simulink model "Solar_Panel_Tracker"  (R2024a)
settings: Solver=VariableStepAuto  StartTime=0.0  StopTime=10.0  RelTol=1e-3
settings Model: Creator=VICTUS  LastModifiedBy=VICTUS

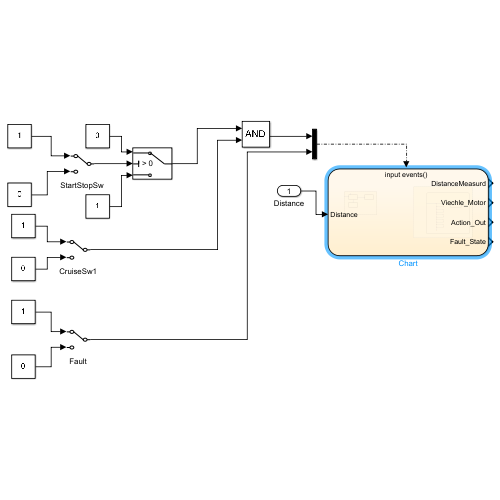
[thumbnail: Simulink's stored preview of the top-level diagram]
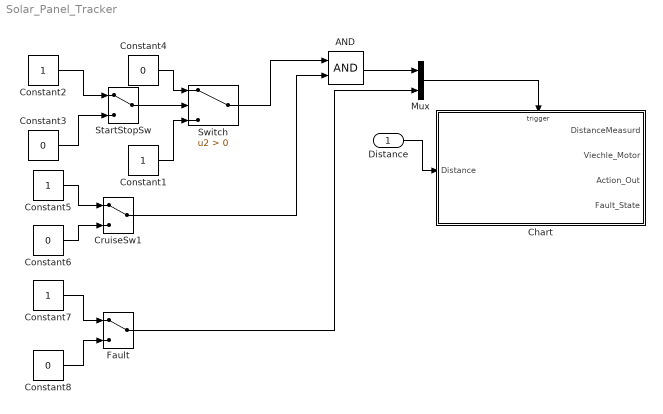
== system Solar_Panel_Tracker ==
  Distance : Inport
  AND : Logic  AllPortsSameDT=off  OutDataTypeStr=boolean
  Chart : Stateflow chart  TreatAsAtomicUnit=on
  Constant{1..2,5,7} (4 alike) : Constant
  Constant{3..4,6,8} (4 alike) : Constant  Value=0
  CruiseSw1 : ManualSwitch
  Fault : ManualSwitch
  Mux : Mux  Inputs=2
  StartStopSw : ManualSwitch
  Switch : Switch  Criteria=u2 > Threshold  SaturateOnIntegerOverflow=off  InputSameDT=off
  wires:
  Constant3/1 -> StartStopSw/2
  Constant2/1 -> StartStopSw/1
  StartStopSw/1 -> Switch/2
  Constant4/1 -> Switch/1
  Switch/1 -> AND/1
  Constant6/1 -> CruiseSw1/2
  Constant5/1 -> CruiseSw1/1
  CruiseSw1/1 -> AND/2
  Constant1/1 -> Switch/3
  Distance/1 -> Chart/1(Distance)
  Constant7/1 -> Fault/1
  Constant8/1 -> Fault/2
  Fault/1 -> Mux/2
  Mux/1 -> Chart/Trigger
  AND/1 -> Mux/1

== stateflow chart Solar_Panel_Tracker/Chart ==
  settings: executeAtInitialization=1
  state RegularSystem [parallel]
    settings: executionOrder=2
    state operation_of_cruise_control
      state DistanceMeasurd
        en:
        DistanceMeasurd = 10;
        du:
        DistanceMeasurd = Distance ;
        (history)
      operation_of_cruise_control -> (junction 34) : cruisecontrol
      (junction 34) -> (junction 36) [order 1] : [DistanceMeasurd > 15]
      (junction 34) -> (junction 40) [order 2]
      (junction 36) -> (junction 38) : {Action_Out = 2;}
          | %acclerate
      (junction 38) -> (junction 40)
      (junction 40) -> (junction 43)
      (junction 43) -> (junction 45) [order 1] : [DistanceMeasurd > 10]
      (junction 43) -> (junction 49) [order 2]
      (junction 45) -> (junction 47) : {Action_Out = 3;}
          | %decelrate
      (junction 47) -> (junction 49)
      (junction 49) -> (junction 53)
      (junction 53) -> (junction 55) [order 1] : [DistanceMeasurd > 10&& DistanceMeasurd > 5]
      (junction 53) -> (junction 59) [order 2]
      (junction 55) -> (junction 57) : {Action_Out = 1;}
          | %donothing
      (junction 57) -> (junction 59)
      (junction 59) -> (junction 63)
      (junction 63) -> (junction 65) [order 1] : [DistanceMeasurd < 5]
      (junction 65) -> (junction 67) : {Action_Out = 0;}
          | %brake
      (junction 63) -> (junction 69) [order 2]
      (junction 67) -> (junction 69)
      (junction 69) -> (junction 74)
      (junction 74) -> (junction 76) [order 1] : [DistanceMeasurd < 1.5]
      (junction 74) -> (junction 80) [order 2]
      (junction 76) -> (junction 78) : {Viechle_Motor = 0;}
      (junction 78) -> (junction 80)
      (junction 80) -> (junction 84)
  state FaultDetectionSystem [parallel]
    settings: executionOrder=1
    state FaultTimer
      en:
      Timer = 0;
      du:
      Timer = Timer + 1;
    state Notification
      en:
      Fault_State = 1;
    state Non_Fault
      en:
      Fault_State = 0;
    (default) -> FaultTimer
    FaultDetectionSystem -> FaultTimer : Fault
    FaultTimer -> Notification [order 1] : [Timer == 10;]
    FaultTimer -> Non_Fault [order 2] : [Timer <= 10;]
  data: Distance input double; DistanceMeasurd output double; Viechle_Motor output boolean; Timer local; Action_Out output; Fault_State output
  events: cruisecontrol input FUNCTION_CALL_EVENT; Fault input FUNCTION_CALL_EVENT
